simulink model "ModelE"  (R2014a)
settings: Solver=FixedStepDiscrete  StartTime=0.0  StopTime=10.0  RelTol=1e-3
libraries: simulink x1
settings Model: SimulationMode=external  ExtModeTrigDuration=100  Creator=admin  LastModifiedBy=admin
settings SolverCC: AutoInsertRateTranBlk=on
settings DataIOCC: SaveOutput=off  SaveTime=off
settings OptimizationCC: InlineParams=on  InlineInvariantSignals=on  StateBitsets=on  DataBitsets=on  UseTempVars=on  ZeroExternalMemoryAtStartup=off  ZeroInternalMemoryAtStartup=off  NoFixptDivByZeroProtection=on  EfficientFloat2IntCast=on  OptimizeModelRefInitCode=on  LifeSpan=1
settings DebuggingCC: SolverPrmCheckMsg=none
settings HardwareCC: ProdLargestAtomicInteger=Long  ProdLargestAtomicFloat=Double  ProdEndianess=LittleEndian  ProdHWDeviceType=ARM Compatible->ARM Cortex
settings RTWCC: SystemTargetFile=realtime.tlc  TLCOptions=-p0  GenCodeOnly=on  GenerateMakefile=off  TemplateMakefile=realtime.tmf  Description=Run on Target Hardware  RTWVerbose=off  ProcessScript=realtime_make_rtw_hook  IncludeHyperlinkInReport=on
settings CodeAppCC: ForceParamTrailComments=on  SimulinkDataObjDesc=on  CustomSymbolStrGlobalVar=rt$N$M  CustomSymbolStrType=$N$M  CustomSymbolStrFcn=$N$M$F  CustomSymbolStrMacro=$N$M  InsertBlockDesc=on
settings STFCustomTargetCC: TargetLibSuffix=.a  GenerateSampleERTMain=on  ConcurrentExecutionCompliant=off  GeneratePreprocessorConditionals=Use local settings  ERTCustomFileBanners=on  SupportNonInlinedSFcns=off  SupportVariableSizeSignals=on  MATLABClassNameForMDSCustomization=Simulink.SoftwareTarget.ERTCustomization  GRTInterface=off  SystemTargetFile=realtime.tlc
settings ERTTargetCC: CombineOutputUpdateFcns=off  SupportContinuousTime=on  SupportVariableSizeSignals=on  ExtModeMexArgs='localhost' 0 17725  ERTSrcFileBannerTemplate=realtime_code_template.cgt  ERTHdrFileBannerTemplate=realtime_code_template.cgt  ERTDataSrcFileTemplate=realtime_code_template.cgt  ERTDataHdrFileTemplate=realtime_code_template.cgt  ERTCustomFileTemplate=realtime_file_process.tlc

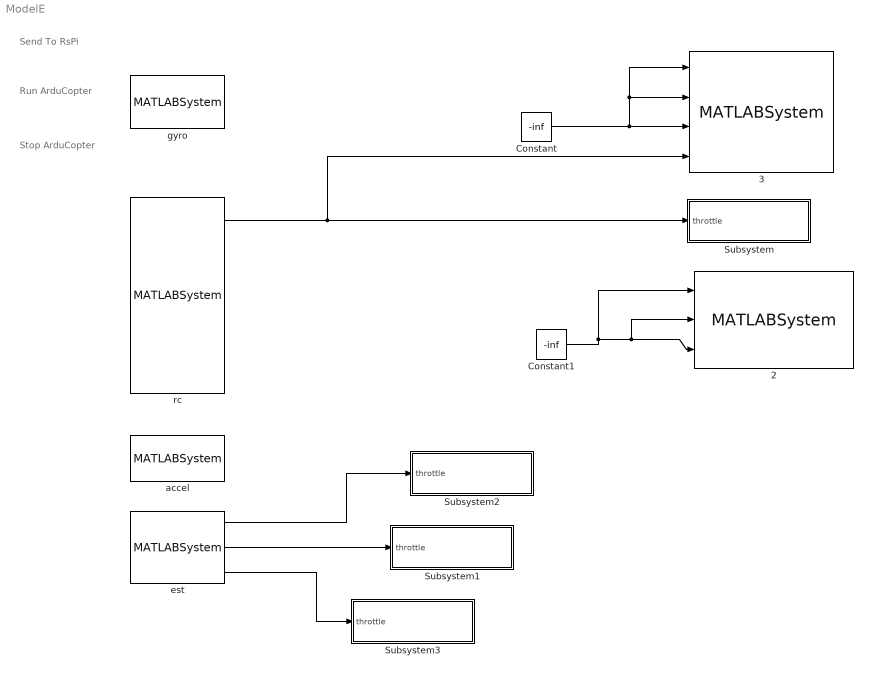
== system ModelE ==
  note: Send To RsPi
  note: Run ArduCopter
  note: Stop ArduCopter
  "   2" : MATLABSystem  System=RateController  SimulateUsing=Interpreted execution
      mask Type: RateController
      mask Display:
      | disp('RateController');
      | port_label('input',1,'yaw');
      | port_label('input',2,'pitch');
      | port_label('input',3,'roll');
  "   3" : MATLABSystem  System=Motors  SimulateUsing=Interpreted execution
      mask Type: Motors
      mask Display:
      | disp('Motors');
      | port_label('input',1,'roll');
      | port_label('input',2,'pitch');
      | port_label('input',3,'yaw');
      | port_label('input',4,'throttle');
  "   rc" : MATLABSystem  System=RC  SimulateUsing=Interpreted execution
      mask Type: RC
      mask Display:
      | disp('RC');
      | port_label('output',1,'thort');
      | port_label('output',2,'yawR');
      | port_label('output',3,'pitch');
      | port_label('output',4,'roll');
  "  accel " : MATLABSystem  System=Accel  SimulateUsing=Interpreted execution
      mask Type: Accel
      mask Display:
      | disp('Accel');
      | port_label('output',1,'x');
      | port_label('output',2,'y');
      | port_label('output',3,'z');
  "  est" : MATLABSystem  System=Copter_Self_State  SimulateUsing=Interpreted execution
      mask Type: Copter_Self_State
      mask Display:
      | disp('Copter_Self_State');
      | port_label('output',1,'yaw');
      | port_label('output',2,'roll');
      | port_label('output',3,'pitch');
  Constant : Constant  Value=-inf
  Constant1 : Constant  Value=-inf
  Subsystem : Subsystem
      mask Display: fprintf('Check throttle range')
  Subsystem1 : Subsystem
      mask Display: fprintf('Check throttle range')
  Subsystem2 : Subsystem
      mask Display: fprintf('Check throttle range')
  Subsystem3 : Subsystem
      mask Display: fprintf('Check throttle range')
  "gyro  " : MATLABSystem  System=Gyro  SimulateUsing=Interpreted execution
      mask Type: Gyro
      mask Display:
      | disp('Gyro');
      | port_label('output',1,'x');
      | port_label('output',2,'y');
      | port_label('output',3,'z');
  wires:
  Constant/1 -> "   3"/2, "   3"/1, "   3"/3
  "   rc"/1 -> "   3"/4, Subsystem/1(throttle)
  Constant1/1 -> "   2"/1, "   2"/2, "   2"/3
  "  est"/2 -> Subsystem1/1(throttle)
  "  est"/1 -> Subsystem2/1(throttle)
  "  est"/3 -> Subsystem3/1(throttle)

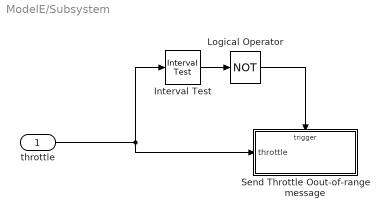
== system ModelE/Subsystem ==
  throttle : Inport
  Interval Test : simulink/Logic and Bit Operations/Interval Test  IntervalClosedRight=on  uplimit=0  IntervalClosedLeft=on  lowlimit=1000  OutDataTypeStr=boolean
  Logical Operator : Logic  Operator=NOT  AllPortsSameDT=off  OutDataTypeStr=boolean
  Send Throttle Oout-of-range message : Subsystem  TreatAsAtomicUnit=on
  wires:
  throttle/1 -> Interval Test/1, Send Throttle Oout-of-range message/1(throttle)
  Logical Operator/1 -> Send Throttle Oout-of-range message/Trigger
  Interval Test/1 -> Logical Operator/1

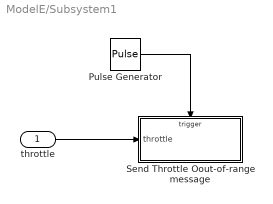
== system ModelE/Subsystem1 ==
  throttle : Inport
  Pulse Generator : DiscretePulseGenerator  Period=100  SampleTime=-1
  Send Throttle Oout-of-range message : Subsystem  TreatAsAtomicUnit=on
  wires:
  throttle/1 -> Send Throttle Oout-of-range message/1(throttle)
  Pulse Generator/1 -> Send Throttle Oout-of-range message/Trigger

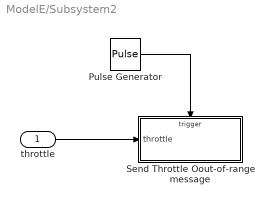
== system ModelE/Subsystem2 ==
  throttle : Inport
  Pulse Generator : DiscretePulseGenerator  Period=100  SampleTime=-1
  Send Throttle Oout-of-range message : Subsystem  TreatAsAtomicUnit=on
  wires:
  Pulse Generator/1 -> Send Throttle Oout-of-range message/Trigger
  throttle/1 -> Send Throttle Oout-of-range message/1(throttle)

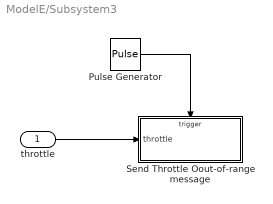
== system ModelE/Subsystem3 ==
  throttle : Inport
  Pulse Generator : DiscretePulseGenerator  Period=100  SampleTime=-1
  Send Throttle Oout-of-range message : Subsystem  TreatAsAtomicUnit=on
  wires:
  Pulse Generator/1 -> Send Throttle Oout-of-range message/Trigger
  throttle/1 -> Send Throttle Oout-of-range message/1(throttle)

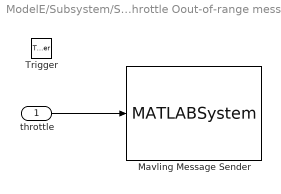
== system ModelE/Subsystem/Send Throttle Oout-of-range message ==
  throttle : Inport
  Trigger : TriggerPort
  Mavling Message Sender : MATLABSystem  System=MavlinkMsg  Message=throttle not between 0 to 1:
      mask Type: MavlinkMsg
      mask Display:
      | disp('MavlinkMsg');
      | port_label('input',1,'u');
  wires:
  throttle/1 -> Mavling Message Sender/1

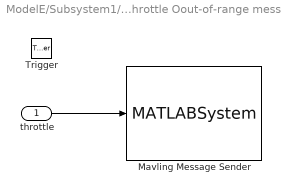
== system ModelE/Subsystem1/Send Throttle Oout-of-range message ==
  throttle : Inport
  Trigger : TriggerPort
  Mavling Message Sender : MATLABSystem  System=MavlinkMsg  Message=estimated roll:
      mask Type: MavlinkMsg
      mask Display:
      | disp('MavlinkMsg');
      | port_label('input',1,'u');
  wires:
  throttle/1 -> Mavling Message Sender/1

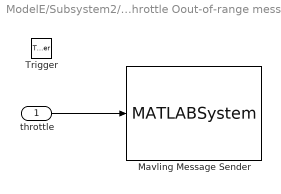
== system ModelE/Subsystem2/Send Throttle Oout-of-range message ==
  throttle : Inport
  Trigger : TriggerPort
  Mavling Message Sender : MATLABSystem  System=MavlinkMsg  Message=estimated pitch:
      mask Type: MavlinkMsg
      mask Display:
      | disp('MavlinkMsg');
      | port_label('input',1,'u');
  wires:
  throttle/1 -> Mavling Message Sender/1

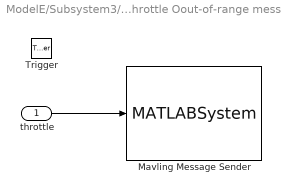
== system ModelE/Subsystem3/Send Throttle Oout-of-range message ==
  throttle : Inport
  Trigger : TriggerPort
  Mavling Message Sender : MATLABSystem  System=MavlinkMsg  Message=estimated pitch:
      mask Type: MavlinkMsg
      mask Display:
      | disp('MavlinkMsg');
      | port_label('input',1,'u');
  wires:
  throttle/1 -> Mavling Message Sender/1
